simulink model "flightSimulation"  (R2018a)
settings: Solver=FixedStepAuto  StartTime=0  StopTime=end_time  FixedStep=0.005  RelTol=1e-3  EnableMultiTasking=on
values from neighbouring files (symbols this model uses):
  initPosLLA = [37.6287386167 -122.393391133 100]    [cmdh.mat]    (also in cmdyaw.mat)
  mass = 1.53    [cmdh.mat]    (also in cmdyaw.mat)
  Ts = 0.01    [cmdh.mat]    (also in cmdyaw.mat)
undefined symbols (not defined in the file or in its folder): B, Earth, ft, m, p_limits, s, sigbuilder_block, sw_turb, umax, umin, Vehicle, WGS84
libraries: simulink x23, aerolibactuator x15, dspswit3 x12, dspsrcs4 x10, dsparch4 x7, aerolibconvert2 x4, aerolibanimutils x2, qcatlib x2, aerolibfltsims x2, aerolibutil x2, shared6dof x1, aerolibtransform2 x1
(part 1 of 4)
settings Model: Creator=The MathWorks, Inc.  LastModifiedBy=mengc
settings SolverCC: AlgebraicLoopSolver=LineSearch  AutoInsertRateTranBlk=on
settings DataIOCC: LimitDataPoints=on  SaveFormat=Array  SaveOutput=off  DSMLogging=off  SaveTime=off
settings OptimizationCC: BlockReduction=off  BufferReuse=off  LifeSpan=inf
settings DebuggingCC: AlgebraicLoopMsg=none  UnderspecifiedInitializationDetection=Classic  MergeDetectMultiDrivingBlocksExec=none  UnconnectedInputMsg=none  UnconnectedOutputMsg=none  UnconnectedLineMsg=none  AllowSymbolicDim=off  SFUnexpectedBacktrackingDiag=warning  SFNoUnconditionalDefaultTransitionDiag=warning  SFExecutionAtInitializationDiag=none
settings HardwareCC: ProdBitPerPointer=32  ProdBitPerSizeT=32  ProdBitPerPtrDiffT=32  ProdLargestAtomicFloat=None  ProdIntDivRoundTo=Undefined  ProdEndianess=Unspecified  ProdWordSize=32  ProdHWDeviceType=32-bit Generic
settings ModelReferenceCC: PropagateSignalLabelsOutOfModel=off
settings CodeAppCC: StateflowObjectComments=on
settings GRTTargetCC: TargetLangStandard=C89/C90 (ANSI)  GeneratePreprocessorConditionals=Disable all
settings ConfigComp: CovMetricSettings=dw  CovHtmlReporting=on  CovSaveCumulativeToWorkspaceVar=on  CovSaveSingleToWorkspaceVar=on  CovExternalEMLEnable=off  CovSFcnEnable=off

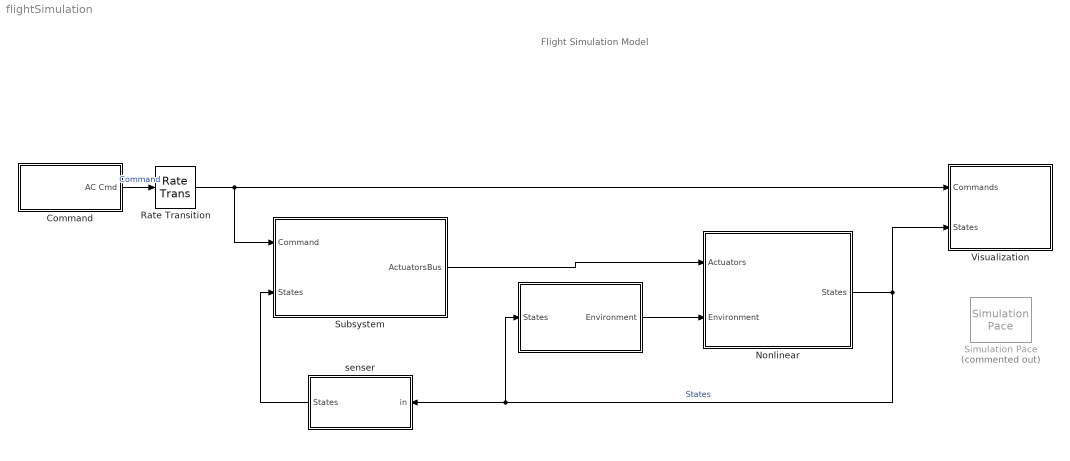
== system flightSimulation ==
  note: Flight Simulation Model
  " " : Subsystem
  Command : Subsystem  Variant=on
  Nonlinear : Subsystem  TreatAsAtomicUnit=on
      mask init:
      | vehicleNonlinearVars;
      settings: MinAlgLoopOccurrences=on
  Rate Transition : RateTransition  OutPortSampleTime=0.01
  Simulation Pace : aerolibanimutils/Simulation Pace  Commented=on  SimulationPace=1  SleepMode=MATLAB Thread  OutputPaceError=off  SampleTime=Ts
      settings: AttributesFormatString=%<SimulationPace> sec/sec
  Subsystem : Subsystem  Variant=on  VariantControl=Variant1
  Visualization : Subsystem
  senser : Subsystem
  wires:
  Nonlinear/1(States) -> senser/1(in), " "/1(States), Visualization/2(States)  "States"
  " "/1(Environment) -> Nonlinear/2(Environment)
  Command/1(AC Cmd) -> Rate Transition/1  "Command"
  Subsystem/1(ActuatorsBus) -> Nonlinear/1(Actuators)
  Rate Transition/1 -> Visualization/1(Commands), Subsystem/1("Command ")
  senser/1(States) -> Subsystem/2(States)

== system flightSimulation/  ==
  States : Inport  OutDataTypeStr=Bus: StatesBus
  Air Density : Constant  Value=1.225
  Air Temp : Constant  Value=273+15
  Bus Creator : BusCreator  Inputs=5  OutDataTypeStr=Bus: EnvironmentBus  NonVirtualBus=on
  Bus Creator1 : BusCreator  Inputs=4  OutDataTypeStr=Bus: AtmosphereBus  NonVirtualBus=on
  Gravity : Constant  Value=[0;0;9.788]
  Magnetic Field : Constant  Value=[0 0 0]
  Memory : Memory  InheritSampleTime=on
  Pressure : Constant  Value=101.3e3
  Speed of Sound : Constant  Value=340
  wind : Constant  Value=[0 0 0]
  Environment : Outport  OutDataTypeStr=Bus: EnvironmentBus
  wires:
  Pressure/1 -> Bus Creator1/3  "pressure"
  Magnetic Field/1 -> Bus Creator/3  "MagneticField_ned"
  Air Density/1 -> Bus Creator1/4  "air_density"
  Bus Creator1/1 -> Bus Creator/2  "AtmosphereBus"
  Gravity/1 -> Bus Creator/1  "Gravity_ned"
  Air Temp/1 -> Bus Creator1/1  "air_temp"
  Speed of Sound/1 -> Bus Creator1/2  "speed_sound"
  wind/1 -> Bus Creator/5  "Wind_ned"
  States/1 -> Memory/1  "StatesBus"
  Bus Creator/1 -> Environment/1  "EnvironmentBus"
  Memory/1 -> Bus Creator/4  "StatesBus"

== system flightSimulation/Command ==
  note: VSS_COMMAND = 0 will select Signal Builder
      | VSS_COMMAND =1 will select Joystick + Signal Builder
      | VSS_COMMAND = 2 will select pre-saved data from .mat file
      | VSS_COMMAND = 3 will select pre-saved data from a spreadsheet
  Data : Subsystem  VariantControl=VSS_COMMAND_PRESAVED
  Joystick : Subsystem  VariantControl=VSS_COMMAND_JOYSTICK
  Signal Builder : Subsystem  VariantControl=VSS_COMMAND_SIGBLDR
  Subsystem : Subsystem  VariantControl=VSS_COMMAND_user
  AC Cmd : Outport  OutDataTypeStr=Bus: CommandBus

== system flightSimulation/Nonlinear ==
  Actuators : Inport  OutDataTypeStr=Bus: ActuatorsBus
  Environment : Inport  Port=2  OutDataTypeStr=Bus: EnvironmentBus
  Plant : Subsystem
  States : Outport
  wires:
  Actuators/1 -> Plant/1(Actuators)  "ActuatorsBus"
  Environment/1 -> Plant/2(Environment)  "Environment"
  Plant/1(States) -> States/1

== system flightSimulation/Subsystem ==
  "Command " : Inport  OutDataTypeStr=Bus: CommandBus
  States : Inport  Port=2  OutDataTypeStr=Bus: StatesBus
  ADRC_allocator : Subsystem  VariantControl=controller==0
  ADRC_allocator1 : Subsystem  VariantControl=controller==1
  PID : Subsystem  VariantControl=controller==2
  PID_allocator : Subsystem  VariantControl=controller==3
  PID_allocator1 : Subsystem  VariantControl=controller==4
  ActuatorsBus : Outport  OutDataTypeStr=Bus: ActuatorsBus

== system flightSimulation/Visualization ==
  Commands : Inport
  States : Inport  Port=2
  Airspeed Indicator : Subsystem  DialogController=aeroblksHMICreateDDGDialog  IsWebBlock=on  mask(MWDashboardBlock){webBlockId=8420f0a9-3312-4f04-a723-760894642590, webBlockType=airspeedindicator, ShowInLibBrowser=on, ShowInitialText=on, HMISrcModelName=flightSimulation}
      mask prompts: webBlockId "WebBlock Id"; webBlockType "WebBlock Type"; HMISrcModelName "Source Model"
      mask help: Display aircraft airspeed in knots.
      mask Help: asbhmihelp('airspeedindicator')
      mask Display:
      | if strcmp(get_param(bdroot(gcb),'BlockDiagramType'), 'library')
      |  image([(matlabroot) '/toolbox/aeroblks/aeroblks/hmi/icons/AirspeedIndicatorIcon.svg'])
      | end
  Altimeter : Subsystem  DialogController=aeroblksHMICreateDDGDialog  IsWebBlock=on  mask(MWDashboardBlock){webBlockId=acc0ee33-6e2a-46f3-b359-bda7f19c378b, webBlockType=altimeter, ShowInLibBrowser=on, ShowInitialText=on, HMISrcModelName=flightSimulation}
      mask prompts: webBlockId "WebBlock Id"; webBlockType "WebBlock Type"; HMISrcModelName "Source Model"
      mask help: Display aircraft altitude in feet.
      mask Help: asbhmihelp('altimeter')
      mask Display:
      | if strcmp(get_param(bdroot(gcb),'BlockDiagramType'), 'library')
      |  image([(matlabroot) '/toolbox/aeroblks/aeroblks/hmi/icons/AltimeterIcon.svg'])
      | end
  Artificial Horizon : Subsystem  DialogController=aeroblksHMICreateDDGDialog  IsWebBlock=on  mask(MWDashboardBlock){webBlockId=e5cf728d-e454-405c-bb84-955fe1273f2a, webBlockType=artificialhorizon, ShowInLibBrowser=on, ShowInitialText=on, HMISrcModelName=flightSimulation}
      mask prompts: webBlockId "WebBlock Id"; webBlockType "WebBlock Type"; HMISrcModelName "Source Model"
      mask help: Display aircraft attitude relative to horizon. The two signal input vector contains roll and pitch.
      mask Help: asbhmihelp('artificialhorizon')
      mask Display:
      | if strcmp(get_param(bdroot(gcb),'BlockDiagramType'), 'library')
      |  image([(matlabroot) '/toolbox/aeroblks/aeroblks/hmi/icons/ArtificialHorizonIcon.svg'])
      | end
  Climb Rate Indicator : Subsystem  DialogController=aeroblksHMICreateDDGDialog  IsWebBlock=on  mask(MWDashboardBlock){webBlockId=da4b646e-398f-4414-b979-eb288c63e8d1, webBlockType=climbindicator, ShowInLibBrowser=on, ShowInitialText=on, HMISrcModelName=flightSimulation}
      mask prompts: webBlockId "WebBlock Id"; webBlockType "WebBlock Type"; HMISrcModelName "Source Model"
      mask help: Display aircraft climb rate in ft/min.
      mask Help: asbhmihelp('climbindicator')
      mask Display:
      | if strcmp(get_param(bdroot(gcb),'BlockDiagramType'), 'library')
      |  image([(matlabroot) '/toolbox/aeroblks/aeroblks/hmi/icons/ClimbIndicatorIcon.svg'])
      | end
  Extract Flight Instruments : Subsystem
  Heading Indicator : Subsystem  DialogController=aeroblksHMICreateDDGDialog  IsWebBlock=on  mask(MWDashboardBlock){webBlockId=33c4a518-f501-4d9d-9c87-ec3702c656b3, webBlockType=headingindicator, ShowInLibBrowser=on, ShowInitialText=on, HMISrcModelName=flightSimulation}
      mask prompts: webBlockId "WebBlock Id"; webBlockType "WebBlock Type"; HMISrcModelName "Source Model"
      mask help: Display aircraft heading with respect to North in degrees.
      mask Help: asbhmihelp('headingindicator')
      mask Display:
      | if strcmp(get_param(bdroot(gcb),'BlockDiagramType'), 'library')
      |  image([(matlabroot) '/toolbox/aeroblks/aeroblks/hmi/icons/HeadingIndicatorIcon.svg'])
      | end
  Visualization : Subsystem  Variant=on
  wires:
  Commands/1 -> Visualization/2(Commands)
  States/1 -> Visualization/1(States), Extract Flight Instruments/1(States)

== system flightSimulation/senser ==
  in : Inport  OutDataTypeStr=Bus: StatesBus
  Bus Creator5 : BusCreator  Inputs=9  OutDataTypeStr=Bus: StatesBus  NonVirtualBus=on
  Bus Selector1 : BusSelector  OutputSignals=V_body,Omega_body,Euler,Accel_body,dOmega_body,V_ned,X_ned,LLA,DCM_be
  Rate Transition2 : RateTransition  OutPortSampleTime=0.01
  noise : Subsystem
  States : Outport  OutDataTypeStr=Bus: StatesBus
  wires:
  Bus Selector1/1 -> Bus Creator5/1  "<V_body>"
  in/1 -> Bus Selector1/1
  Bus Selector1/7 -> Bus Creator5/7  "<X_ned>"
  Bus Selector1/8 -> Bus Creator5/8  "<LLA>"
  Bus Selector1/2 -> Bus Creator5/2  "<Omega_body>"
  Bus Selector1/9 -> Bus Creator5/9  "<DCM_be>"
  Bus Selector1/4 -> Bus Creator5/4  "<Accel_body>"
  Bus Selector1/5 -> Bus Creator5/5  "<dOmega_body>"
  Bus Selector1/6 -> Bus Creator5/6  "<V_ned>"
  Bus Selector1/3 -> noise/1(In1)  "<Euler>"
  Bus Creator5/1 -> Rate Transition2/1
  noise/1(Out1) -> Bus Creator5/3  "Euler"
  Rate Transition2/1 -> States/1

== system flightSimulation/Command/Data ==
  Bus Creator : BusCreator  Inputs=4  OutDataTypeStr=Bus: CommandBus  NonVirtualBus=on
  From Workspace : FromWorkspace  VariableName=cmdroll  SampleTime=0
  From Workspace1 : FromWorkspace  VariableName=cmdpitch  SampleTime=0
  From Workspace2 : FromWorkspace  VariableName=cmdyaw  SampleTime=0
  From Workspace3 : FromWorkspace  VariableName=cmdh  SampleTime=0
  Step : Step  Time=10  After=0.1  SampleTime=0
  Step1 : Step  Time=10  After=0  SampleTime=0
  Terminator : Terminator
  AC Cmd : Outport  OutDataTypeStr=Bus: CommandBus
  wires:
  Bus Creator/1 -> AC Cmd/1
  From Workspace1/1 -> Bus Creator/2  "pitch_cmd"
  From Workspace2/1 -> Bus Creator/3  "yaw_cmd"
  From Workspace3/1 -> Bus Creator/4  "throttle_cmd"
  From Workspace/1 -> Bus Creator/1  "roll_cmd"
  Step/1 -> Terminator/1

== system flightSimulation/Command/Joystick ==
  Bus Creator : BusCreator  Inputs=4  OutDataTypeStr=Bus: CommandBus  NonVirtualBus=on
  Pilot Joystick : aerolibanimutils/Pilot Joystick  JoystickID=Joystick1  OutputConfiguration=FourAxis  SampleTime=Ts
  AC Cmd : Outport  OutDataTypeStr=Bus: CommandBus
  wires:
  Pilot Joystick/4 -> Bus Creator/4  "throttle_cmd"
  Pilot Joystick/3 -> Bus Creator/3  "yaw_cmd"
  Pilot Joystick/2 -> Bus Creator/2  "pitch_cmd"
  Pilot Joystick/1 -> Bus Creator/1  "roll_cmd"
  Bus Creator/1 -> AC Cmd/1

== system flightSimulation/Command/Signal Builder ==
  Bus Creator : BusCreator  Inputs=4  OutDataTypeStr=Bus: CommandBus  NonVirtualBus=on
  N-Sample Switch : dspswit3/N-Sample Switch  N=200  reset=off  TriggerType=Rising edge  Ts=0.01
      settings: SourceProductName=DSP System Toolbox  SourceProductBaseCode=DS
  Pulse Generator : DiscretePulseGenerator  Amplitude=0.2  Period=300  PulseWidth=150  SampleTime=0.01
  Signal Builder : Subsystem  Tag=STV Subsys  LoadFcn=sigbuilder_block('load',[3 6 804 505.5 ]);  StartFcn=sigbuilder_block('start');  StopFcn=sigbuilder_block('stop');  ClipboardFcn=sigbuilder_block('clipboard');  mask(Sigbuilder block){tuvar=[0:10]}
      mask help: Simulink:masks:SigbuilderBlock_MD
      mask init:
      | if ~strcmp(get_param(bdroot(gcbh),'SimulationStatus'),'stopped') tuvar = sigbuilder_block('maskInit'); end
      settings: CopyFcn=sigbuilder_block('copy');  DeleteFcn=sigbuilder_block('delete');  ModelCloseFcn=sigbuilder_block('modelClose');  PreSaveFcn=sigbuilder_block('preSave');  PauseFcn=sigbuilder_block('pause');  ContinueFcn=sigbuilder_block('continue');  NameChangeFcn=sigbuilder_block('namechange');  OpenFcn=sigbuilder_block('open',[3 6 804 505.5 ]);  CloseFcn=sigbuilder_block('close');
      mask Display: plot(0, 0, 100, 100,[2, 2, 32, 32, 2], [68, 8, 8, 68, 68],[32, 2], [38, 38], [32, 19, 2],[53, 60, 44], [32, 17, 17, 2],[16, 16, 31, 31]);txt = getActiveGroup(gcbh);text(2, 100, txt,'verticalAlignment', 'top');
  Sine Wave : Sin  Amplitude=0.2  Frequency=2*pi/3  Samples=2000  SampleTime=0.01
  To Workspace : ToWorkspace  VariableName=simout  SaveFormat=Timeseries  SampleTime=-1
  roll_cmd : Step  Time=0  After=0  SampleTime=0
  throttle_cmd : Step  Time=0  After=0.5  SampleTime=0
  yaw_cmd : Step  Time=0  After=0  SampleTime=0
  AC Cmd : Outport  OutDataTypeStr=Bus: CommandBus
  wires:
  Bus Creator/1 -> AC Cmd/1
  Signal Builder/4(throttle_cmd) -> Bus Creator/4  "throttle_cmd"
  Signal Builder/2(picth_cmd) -> Bus Creator/2  "pitch_cmd"
  Signal Builder/3(yaw_cmd) -> Bus Creator/3  "yaw_cmd"
  Signal Builder/1(roll_cmd) -> Bus Creator/1  "roll_cmd"
  Pulse Generator/1 -> N-Sample Switch/2

== system flightSimulation/Command/Subsystem ==
  Bus Creator : BusCreator  Inputs=4  OutDataTypeStr=Bus: CommandBus  NonVirtualBus=on
  Signal Builder : Subsystem  Tag=STV Subsys  LoadFcn=sigbuilder_block('load',[0 30 1024.5 487.5 ]);  StartFcn=sigbuilder_block('start');  StopFcn=sigbuilder_block('stop');  ClipboardFcn=sigbuilder_block('clipboard');  mask(Sigbuilder block){tuvar=[0:10]}
      mask help: Simulink:masks:SigbuilderBlock_MD
      mask init:
      | if ~strcmp(get_param(bdroot(gcbh),'SimulationStatus'),'stopped') tuvar = sigbuilder_block('maskInit'); end
      settings: CopyFcn=sigbuilder_block('copy');  DeleteFcn=sigbuilder_block('delete');  ModelCloseFcn=sigbuilder_block('modelClose');  PreSaveFcn=sigbuilder_block('preSave');  PauseFcn=sigbuilder_block('pause');  ContinueFcn=sigbuilder_block('continue');  NameChangeFcn=sigbuilder_block('namechange');  OpenFcn=sigbuilder_block('open',[3 6 804 505.5 ]);  CloseFcn=sigbuilder_block('close');
      mask Display: plot(0, 0, 100, 100,[2, 2, 32, 32, 2], [68, 8, 8, 68, 68],[32, 2], [38, 38], [32, 19, 2],[53, 60, 44], [32, 17, 17, 2],[16, 16, 31, 31]);txt = getActiveGroup(gcbh);text(2, 100, txt,'verticalAlignment', 'top');
  Signal Builder1 : Subsystem  Tag=STV Subsys  LoadFcn=sigbuilder_block('load');  StartFcn=sigbuilder_block('start');  StopFcn=sigbuilder_block('stop');  ClipboardFcn=sigbuilder_block('clipboard');  mask(Sigbuilder block){tuvar=[0:10]}
      mask help: Simulink:masks:SigbuilderBlock_MD
      mask init:
      | if ~strcmp(get_param(bdroot(gcbh),'SimulationStatus'),'stopped') tuvar = sigbuilder_block('maskInit'); end
      settings: CopyFcn=sigbuilder_block('copy');  DeleteFcn=sigbuilder_block('delete');  ModelCloseFcn=sigbuilder_block('modelClose');  PreSaveFcn=sigbuilder_block('preSave');  PauseFcn=sigbuilder_block('pause');  ContinueFcn=sigbuilder_block('continue');  NameChangeFcn=sigbuilder_block('namechange');  OpenFcn=sigbuilder_block('open',[0 30 1024.5 487.5 ]);  CloseFcn=sigbuilder_block('close');
      mask Display: plot(0, 0, 100, 100,[2, 2, 32, 32, 2], [68, 8, 8, 68, 68],[32, 2], [38, 38], [32, 19, 2],[53, 60, 44], [32, 17, 17, 2],[16, 16, 31, 31]);txt = getActiveGroup(gcbh);text(2, 100, txt,'verticalAlignment', 'top');
  AC Cmd : Outport  OutDataTypeStr=Bus: CommandBus
  wires:
  Bus Creator/1 -> AC Cmd/1
  Signal Builder/1(roll_cmd) -> Bus Creator/1  "roll_cmd"
  Signal Builder/2(picth_cmd) -> Bus Creator/2  "pitch_cmd"
  Signal Builder/3(yaw_cmd) -> Bus Creator/3  "yaw_cmd"
  Signal Builder/4(throttle_cmd) -> Bus Creator/4  "throttle_cmd"

== system flightSimulation/Nonlinear/Plant ==
  Actuators : Inport  OutDataTypeStr=Bus: ActuatorsBus
  Environment : Inport  Port=2  OutDataTypeStr=Bus: EnvironmentBus
  6DOF (Quaternion) : shared6dof/6DOF (Euler Angles)  units=Metric (MKS)  mtype=Fixed  rep=Euler Angles  xme_0=initPosNED  Vm_0=initVb  eul_0=initEuler  pm_0=initAngRates  mass_0=mass  mass_e=0.5  mass_f=2.0  inertia=inertia  inertia_e=eye(3)  inertia_f=2*eye(3)  k_quat=Vehicle.Nonlinear.Nonlinear.SixDOF.quatGain  vre_flag=on  abi_flag=on  aMode=aMode
      settings: SourceProductBaseCode=AE
  Bus setup : Subsystem
  Position on Earth : Subsystem  Priority=1  TreatAsAtomicUnit=on
  Subsystem : Subsystem
  Subsystem1 : Subsystem
  Sum : Sum  Inputs=|++
  Terminator : Terminator
  States : Outport  OutDataTypeStr=Bus: StatesBus
  wires:
  Position on Earth/1(LLA) -> Bus setup/1(LLA)
  6DOF (Quaternion)/8 -> Terminator/1
  6DOF (Quaternion)/1 -> Bus setup/2(V_ned)
  6DOF (Quaternion)/2 -> Position on Earth/1(Xe), Bus setup/3(X_ned)
  6DOF (Quaternion)/9 -> Bus setup/9(Accel_b)
  6DOF (Quaternion)/5 -> Bus setup/6(V_b)
  6DOF (Quaternion)/7 -> Bus setup/8(dOmega_b)
  6DOF (Quaternion)/4 -> Bus setup/5(DCM_be)  "Rn2b"
  Bus setup/1(States) -> States/1  "StatesBus"
  Environment/1 -> Subsystem/2(EnvironmentBus), Subsystem1/2(In2)  "EnvironmentBus"
  Subsystem/1(Out1) -> 6DOF (Quaternion)/1
  Actuators/1 -> Subsystem1/1(In1), Subsystem/1(ActuatorsBus)  "ActuatorsBus"
  Subsystem1/1(Out1) -> Sum/1
  Sum/1 -> 6DOF (Quaternion)/2
  6DOF (Quaternion)/6 -> Bus setup/7(Omega_b)
  6DOF (Quaternion)/3 -> Bus setup/4(Euler)

== system flightSimulation/Subsystem/ADRC_allocator ==
  Command : Inport
  States : Inport  Port=2  OutDataTypeStr=Bus: StatesBus
  Add : Sum
  Bus Creator : BusCreator  Inputs=5  OutDataTypeStr=Bus: ActuatorsBus
  Bus Selector : BusSelector  OutputSignals=roll_cmd,pitch_cmd,yaw_cmd,throttle_cmd
  Bus Selector1 : BusSelector  OutputSignals=<Euler>,Omega_body,X_ned,V_ned
  Constant : Constant  Value=-9.788
  Constant1 : Constant  Value=1225
  Demux : Demux  Outputs=3
  Demux2 : Demux  Outputs=3
  Demux3 : Demux  Outputs=3
  Demux4 : Demux  Outputs=2
  Demux5 : Demux  Outputs=2
  MATLAB Function : MATLAB Function  TreatAsAtomicUnit=on
  MATLAB Function2 : MATLAB Function  TreatAsAtomicUnit=on
  MATLAB Function3 : MATLAB Function  TreatAsAtomicUnit=on
  N-Sample Switch : dspswit3/N-Sample Switch  N=3  reset=off  TriggerType=Rising edge  Ts=0.01
      settings: SourceProductName=DSP System Toolbox  SourceProductBaseCode=DS
  PID Controller (2DOF)7 : simulink/Continuous/PID Controller (2DOF)  Controller=PID  TimeDomain=Discrete-time  SampleTime=-1  IntegratorMethod=Forward Euler  FilterMethod=Forward Euler  Form=Parallel  UseFilter=on  ControllerParametersSource=internal  P=2.1  I=0.2  D=2.1  N=100  b=1  c=1  InitialConditionSource=internal  InitialConditionForIntegrator=0  InitialConditionForFilter=0  ExternalReset=none  LimitOutput=off  UpperSaturationLimit=inf  LowerSaturationLimit=-inf  LinearizeAsGain=on  AntiWindupMode=none  Kb=1  TrackingMode=off  Kt=1  PParamMin=[]  PParamMax=[]  IParamMin=[]  IParamMax=[]  DParamMin=[]  DParamMax=[]  NParamMin=[]  NParamMax=[]  bParamMin=[]  bParamMax=[]  cParamMin=[]  cParamMax=[]  KbParamMin=[]  KbParamMax=[]  KtParamMin=[]  KtParamMax=[]  POutMin=[]  POutMax=[]  IOutMin=[]  IOutMax=[]  DOutMin=[]  DOutMax=[]  NOutMin=[]  NOutMax=[]  bOutMin=[]  bOutMax=[]  cOutMin=[]  cOutMax=[]  KbOutMin=[]  KbOutMax=[]  KtOutMin=[]  KtOutMax=[]  IntegratorOutMin=[]  IntegratorOutMax=[]  FilterOutMin=[]  FilterOutMax=[]  SumOutMin=[]  SumOutMax=[]  Sum1OutMin=[]  Sum1OutMax=[]  Sum2OutMin=[]  Sum2OutMax=[]  Sum3OutMin=[]  Sum3OutMax=[]  SumI1OutMin=[]  SumI1OutMax=[]  SumI2OutMin=[]  SumI2OutMax=[]  SumI3OutMin=[]  SumI3OutMax=[]  SumDOutMin=[]  SumDOutMax=[]  SaturationOutMin=[]  SaturationOutMax=[]  IntegratorContinuousStateAttributes=''  IntegratorStateMustResolveToSignalObject=off  IntegratorRTWStateStorageClass=Auto  FilterContinuousStateAttributes=''  FilterStateMustResolveToSignalObject=off  FilterRTWStateStorageClass=Auto  DifferentiatorICPrevScaledInput=0  DifferentiatorOutMin=[]  DifferentiatorOutMax=[]  FilterDiffOutCoefMin=[]  FilterDiffOutCoefMax=[]  SumDenOutMin=[]  SumDenOutMax=[]  SumNumOutMin=[]  SumNumOutMax=[]  ReciprocalOutMin=[]  ReciprocalOutMax=[]  DivideOutMin=[]  DivideOutMax=[]  TunerSelectOption=Transfer Function Based (PID Tuner App)
  S-Function : S-Function  FunctionName=s_yawTD  SFunctionDeploymentMode=off  EnableBusSupport=off
  S-Function1 : S-Function  FunctionName=s_TD  SFunctionDeploymentMode=off  EnableBusSupport=off
  S-Function2 : S-Function  FunctionName=s_TD  SFunctionDeploymentMode=off  EnableBusSupport=off
  Saturation : Saturate  UpperLimit=9.788  LowerLimit=-9.788
  Subsystem : Subsystem
  Subsystem2 : Subsystem
  TD : Demux  Outputs=2
  Terminator2 : Terminator
  Terminator3 : Terminator
  Unit Delay1 : UnitDelay  SampleTime=-1
  舵机偏角输入eso : Subsystem
  ActuatorsBus : Outport  OutDataTypeStr=Bus: ActuatorsBus
  wires:
  PID Controller (2DOF)7/1 -> Saturation/1
  Bus Selector1/2 -> 舵机偏角输入eso/6(<pqr>)  "<Omega_body>"
  Demux3/2 -> Terminator2/1
  Demux/2 -> Subsystem/1(q)
  Demux3/1 -> Terminator3/1
  Bus Selector/4 -> PID Controller (2DOF)7/1  "<throttle_cmd>"
  Command/1 -> Bus Selector/1
  Bus Creator/1 -> ActuatorsBus/1  "ActuatorsBus"
  Constant1/1 -> N-Sample Switch/1
  Subsystem/1(speed) -> N-Sample Switch/2  "speed"
  N-Sample Switch/1 -> Bus Creator/5  "speed"
  Demux3/3 -> PID Controller (2DOF)7/2  "h"
  States/1 -> Unit Delay1/1
  Unit Delay1/1 -> Bus Selector1/1
  Add/1 -> Subsystem/3(In3)  "a_t"
  Constant/1 -> Add/1
  Saturation/1 -> Add/2
  Demux/1 -> Subsystem/2(p)
  Subsystem2/1(c1) -> Bus Creator/1
  Subsystem2/3(c3) -> Bus Creator/3
  Subsystem2/2(c2) -> Bus Creator/2
  Bus Selector1/3 -> Demux3/1  "<X_ned>"
  Subsystem2/4(c4) -> Bus Creator/4
  Bus Selector1/1 -> 舵机偏角输入eso/5(<Euler>), Demux/1  "<<Euler>>"
  舵机偏角输入eso/7(反馈) -> Demux2/1
  S-Function/1 -> Demux4/1
  Demux4/1 -> MATLAB Function/1(x1_d)  "偏航_跟踪"
  Demux4/2 -> MATLAB Function/2(x2_d)
  Bus Selector/3 -> S-Function/1  "<yaw_cmd>"
  S-Function1/1 -> Demux5/1
  Demux5/2 -> MATLAB Function2/2(x2_d)
  Demux5/1 -> MATLAB Function2/1(x1_d)  "俯仰_跟踪"
  TD/1 -> MATLAB Function3/1(x1_d)  "滚转_跟踪"
  TD/2 -> MATLAB Function3/2(x2_d)
  S-Function2/1 -> TD/1
  Bus Selector/1 -> S-Function2/1  "<roll_cmd>"
  Bus Selector/2 -> S-Function1/1  "<pitch_cmd>"
  MATLAB Function/1(u_r) -> Subsystem2/3(u_3)  "ur"
  MATLAB Function3/1(u_p) -> Subsystem2/1(u_1)  "up"
  MATLAB Function2/1(u_q) -> Subsystem2/2(u_2)  "uq"
  舵机偏角输入eso/1(滚转估计) -> MATLAB Function3/3(x1)
  舵机偏角输入eso/2(俯仰估计) -> MATLAB Function2/3(x1)
  舵机偏角输入eso/3(偏航估计) -> MATLAB Function/3(x1)
  舵机偏角输入eso/4(P估计) -> MATLAB Function3/4(x2)
  舵机偏角输入eso/5(q估计) -> MATLAB Function2/4(x2)
  舵机偏角输入eso/6(r估计) -> MATLAB Function/4(x2)
  Demux2/1 -> Subsystem2/4(u_4)  "dp"
  Demux2/2 -> Subsystem2/5(u_5)  "dq"
  Demux2/3 -> Subsystem2/6(u_6)  "dr"
  Subsystem2/5(c5) -> 舵机偏角输入eso/1(c1)
  Subsystem2/6(c6) -> 舵机偏角输入eso/2(c2)
  Subsystem2/7(c7) -> 舵机偏角输入eso/3(c3)
  Subsystem2/8(c8) -> 舵机偏角输入eso/4(c4)

== system flightSimulation/Subsystem/ADRC_allocator1 ==
  Command : Inport
  States : Inport  Port=2  OutDataTypeStr=Bus: StatesBus
  Add : Sum
  Bus Creator : BusCreator  Inputs=5  OutDataTypeStr=Bus: ActuatorsBus
  Bus Selector : BusSelector  OutputSignals=roll_cmd,pitch_cmd,yaw_cmd,throttle_cmd
  Bus Selector1 : BusSelector  OutputSignals=Euler,Omega_body,X_ned
  Constant : Constant  Value=-9.788
  Constant1 : Constant  Value=1225  SampleTime=0.005
  Demux : Demux  Outputs=3
  Demux2 : Demux  Outputs=3
  Demux3 : Demux  Outputs=3
  Demux4 : Demux  Outputs=2
  Demux5 : Demux  Outputs=2
  MATLAB Function : MATLAB Function  TreatAsAtomicUnit=on
  MATLAB Function2 : MATLAB Function  TreatAsAtomicUnit=on
  MATLAB Function3 : MATLAB Function  TreatAsAtomicUnit=on
  N-Sample Switch : dspswit3/N-Sample Switch  N=10  reset=off  TriggerType=Rising edge  Ts=0.005
      settings: SourceProductName=DSP System Toolbox  SourceProductBaseCode=DS
  PID Controller (2DOF)7 : simulink/Continuous/PID Controller (2DOF)  Controller=PID  TimeDomain=Discrete-time  SampleTime=0.01  IntegratorMethod=Forward Euler  FilterMethod=Forward Euler  Form=Parallel  UseFilter=on  ControllerParametersSource=internal  P=2.1  I=0.2  D=2.1  N=100  b=1  c=1  InitialConditionSource=internal  InitialConditionForIntegrator=0  InitialConditionForFilter=0  ExternalReset=none  LimitOutput=off  UpperSaturationLimit=inf  LowerSaturationLimit=-inf  LinearizeAsGain=on  AntiWindupMode=none  Kb=1  TrackingMode=off  Kt=1  PParamMin=[]  PParamMax=[]  IParamMin=[]  IParamMax=[]  DParamMin=[]  DParamMax=[]  NParamMin=[]  NParamMax=[]  bParamMin=[]  bParamMax=[]  cParamMin=[]  cParamMax=[]  KbParamMin=[]  KbParamMax=[]  KtParamMin=[]  KtParamMax=[]  POutMin=[]  POutMax=[]  IOutMin=[]  IOutMax=[]  DOutMin=[]  DOutMax=[]  NOutMin=[]  NOutMax=[]  bOutMin=[]  bOutMax=[]  cOutMin=[]  cOutMax=[]  KbOutMin=[]  KbOutMax=[]  KtOutMin=[]  KtOutMax=[]  IntegratorOutMin=[]  IntegratorOutMax=[]  FilterOutMin=[]  FilterOutMax=[]  SumOutMin=[]  SumOutMax=[]  Sum1OutMin=[]  Sum1OutMax=[]  Sum2OutMin=[]  Sum2OutMax=[]  Sum3OutMin=[]  Sum3OutMax=[]  SumI1OutMin=[]  SumI1OutMax=[]  SumI2OutMin=[]  SumI2OutMax=[]  SumI3OutMin=[]  SumI3OutMax=[]  SumDOutMin=[]  SumDOutMax=[]  SaturationOutMin=[]  SaturationOutMax=[]  IntegratorContinuousStateAttributes=''  IntegratorStateMustResolveToSignalObject=off  IntegratorRTWStateStorageClass=Auto  FilterContinuousStateAttributes=''  FilterStateMustResolveToSignalObject=off  FilterRTWStateStorageClass=Auto  DifferentiatorICPrevScaledInput=0  DifferentiatorOutMin=[]  DifferentiatorOutMax=[]  FilterDiffOutCoefMin=[]  FilterDiffOutCoefMax=[]  SumDenOutMin=[]  SumDenOutMax=[]  SumNumOutMin=[]  SumNumOutMax=[]  ReciprocalOutMin=[]  ReciprocalOutMax=[]  DivideOutMin=[]  DivideOutMax=[]  TunerSelectOption=Transfer Function Based (PID Tuner App)
  S-Function : S-Function  FunctionName=s_yawTD  SFunctionDeploymentMode=off  EnableBusSupport=off
  S-Function1 : S-Function  FunctionName=s_TD  SFunctionDeploymentMode=off  EnableBusSupport=off
  S-Function2 : S-Function  FunctionName=s_TD  SFunctionDeploymentMode=off  EnableBusSupport=off
  Saturation : Saturate  UpperLimit=9.788  LowerLimit=-9.788
  Subsystem : Subsystem
  Subsystem2 : Subsystem
  TD : Demux  Outputs=2
  Terminator2 : Terminator
  Terminator3 : Terminator
  input noise : Subsystem
  舵机偏角输入eso : Subsystem
  ActuatorsBus : Outport  OutDataTypeStr=Bus: ActuatorsBus
  wires:
  PID Controller (2DOF)7/1 -> Saturation/1
  Bus Selector1/2 -> 舵机偏角输入eso/3(<pqr>)  "<Omega_body>"
  Demux3/2 -> Terminator2/1
  Demux/2 -> Subsystem/1(q)
  Demux3/1 -> Terminator3/1
  Bus Selector/4 -> PID Controller (2DOF)7/1  "<throttle_cmd>"
  Command/1 -> Bus Selector/1
  Bus Creator/1 -> ActuatorsBus/1  "ActuatorsBus"
  Constant1/1 -> N-Sample Switch/1
  Subsystem/1(speed) -> N-Sample Switch/2  "speed"
  N-Sample Switch/1 -> Bus Creator/5  "speed"
  Demux3/3 -> PID Controller (2DOF)7/2  "h"
  Add/1 -> Subsystem/3(In3)  "a_t"
  Constant/1 -> Add/1
  Saturation/1 -> Add/2
  Demux/1 -> Subsystem/2(p)
  Subsystem2/1(c1) -> Bus Creator/1
  Subsystem2/3(c3) -> Bus Creator/3
  Subsystem2/2(c2) -> Bus Creator/2
  Bus Selector1/3 -> Demux3/1  "<X_ned>"
  Subsystem2/4(c4) -> Bus Creator/4
  S-Function/1 -> Demux4/1
  Demux4/1 -> MATLAB Function/1(x1_d)  "偏航_跟踪"
  Demux4/2 -> MATLAB Function/2(x2_d)
  Bus Selector/3 -> input noise/3(In3)  "<yaw_cmd>"
  S-Function1/1 -> Demux5/1
  Demux5/2 -> MATLAB Function2/2(x2_d)
  Demux5/1 -> MATLAB Function2/1(x1_d)  "俯仰_跟踪"
  TD/1 -> MATLAB Function3/1(x1_d)  "滚转_跟踪"
  TD/2 -> MATLAB Function3/2(x2_d)
  S-Function2/1 -> TD/1
  Bus Selector/1 -> input noise/1(In1)  "<roll_cmd>"
  Bus Selector/2 -> input noise/2(In2)  "<pitch_cmd>"
  MATLAB Function/1(u_r) -> Subsystem2/3(u_3)  "ur"
  MATLAB Function3/1(u_p) -> Subsystem2/1(u_1)  "up"
  MATLAB Function2/1(u_q) -> Subsystem2/2(u_2)  "uq"
  舵机偏角输入eso/1(滚转估计) -> MATLAB Function3/3(x1)
  舵机偏角输入eso/2(俯仰估计) -> MATLAB Function2/3(x1)
  舵机偏角输入eso/3(偏航估计) -> MATLAB Function/3(x1)
  舵机偏角输入eso/4(P估计) -> MATLAB Function3/4(x2)
  舵机偏角输入eso/5(q估计) -> MATLAB Function2/4(x2)
  舵机偏角输入eso/6(r估计) -> MATLAB Function/4(x2)
  Demux2/1 -> Subsystem2/4(u_4)  "dp"
  Demux2/2 -> Subsystem2/5(u_5)  "dq"
  Demux2/3 -> Subsystem2/6(u_6)  "dr"
  Subsystem2/5(c5) -> 舵机偏角输入eso/1(c1)
  舵机偏角输入eso/7(反馈) -> Demux2/1
  States/1 -> Bus Selector1/1
  Bus Selector1/1 -> Demux/1, 舵机偏角输入eso/2(<Euler>)  "<Euler>"
  input noise/1(Out1) -> S-Function2/1
  input noise/2(Out2) -> S-Function1/1
  input noise/3(Out3) -> S-Function/1

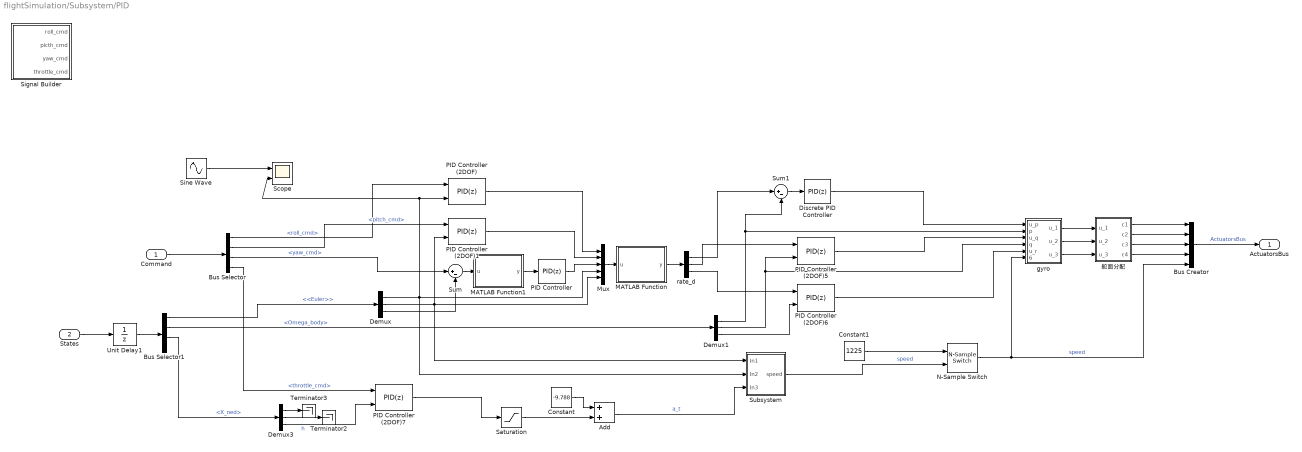
== system flightSimulation/Subsystem/PID ==
  Command : Inport
  States : Inport  Port=2  OutDataTypeStr=Bus: StatesBus
  Add : Sum
  Bus Creator : BusCreator  Inputs=5  OutDataTypeStr=Bus: ActuatorsBus
  Bus Selector : BusSelector  OutputSignals=roll_cmd,pitch_cmd,yaw_cmd,throttle_cmd
  Bus Selector1 : BusSelector  OutputSignals=<Euler>,Omega_body,X_ned,V_ned
  Constant : Constant  Value=-9.788
  Constant1 : Constant  Value=1225
  Demux : Demux  Outputs=3
  Demux1 : Demux  Outputs=3
  Demux3 : Demux  Outputs=3
  Discrete PID Controller : simulink/Continuous/PID Controller  Controller=PID  TimeDomain=Discrete-time  SampleTime=-1  IntegratorMethod=Forward Euler  FilterMethod=Forward Euler  Form=Parallel  UseFilter=on  ControllerParametersSource=internal  P=0.4  I=0.1  D=0  N=100  InitialConditionSource=internal  InitialConditionForIntegrator=0  InitialConditionForFilter=0  ExternalReset=none  LimitOutput=off  UpperSaturationLimit=inf  LowerSaturationLimit=-inf  LinearizeAsGain=off  AntiWindupMode=none  Kb=1  TrackingMode=off  Kt=1  PParamMin=[]  PParamMax=[]  IParamMin=[]  IParamMax=[]  DParamMin=[]  DParamMax=[]  NParamMin=[]  NParamMax=[]  KbParamMin=[]  KbParamMax=[]  KtParamMin=[]  KtParamMax=[]  POutMin=[]  POutMax=[]  IOutMin=[]  IOutMax=[]  DOutMin=[]  DOutMax=[]  NOutMin=[]  NOutMax=[]  KbOutMin=[]  KbOutMax=[]  KtOutMin=[]  KtOutMax=[]  IntegratorOutMin=[]  IntegratorOutMax=[]  FilterOutMin=[]  FilterOutMax=[]  SumOutMin=[]  SumOutMax=[]  SumI1OutMin=[]  SumI1OutMax=[]  SumI2OutMin=[]  SumI2OutMax=[]  SumI3OutMin=[]  SumI3OutMax=[]  SumDOutMin=[]  SumDOutMax=[]  SaturationOutMin=[]  SaturationOutMax=[]  IntegratorContinuousStateAttributes=''  IntegratorStateMustResolveToSignalObject=off  IntegratorRTWStateStorageClass=Auto  FilterContinuousStateAttributes=''  FilterStateMustResolveToSignalObject=off  FilterRTWStateStorageClass=Auto  DifferentiatorICPrevScaledInput=0  DifferentiatorOutMin=[]  DifferentiatorOutMax=[]  FilterDiffOutCoefMin=[]  FilterDiffOutCoefMax=[]  SumDenOutMin=[]  SumDenOutMax=[]  SumNumOutMin=[]  SumNumOutMax=[]  ReciprocalOutMin=[]  ReciprocalOutMax=[]  DivideOutMin=[]  DivideOutMax=[]  TunerSelectOption=Transfer Function Based (PID Tuner App)
  MATLAB Function : MATLAB Function  TreatAsAtomicUnit=on
  MATLAB Function1 : MATLAB Function  TreatAsAtomicUnit=on
  Mux : Mux  Inputs=5
  N-Sample Switch : dspswit3/N-Sample Switch  N=3  reset=off  TriggerType=Rising edge  Ts=0.01
      settings: SourceProductName=DSP System Toolbox  SourceProductBaseCode=DS
  PID Controller : simulink/Continuous/PID Controller  Controller=PID  TimeDomain=Discrete-time  SampleTime=-1  IntegratorMethod=Forward Euler  FilterMethod=Forward Euler  Form=Parallel  UseFilter=on  ControllerParametersSource=internal  P=5  I=0  D=0  N=100  InitialConditionSource=internal  InitialConditionForIntegrator=0  InitialConditionForFilter=0  ExternalReset=none  LimitOutput=off  UpperSaturationLimit=inf  LowerSaturationLimit=-inf  LinearizeAsGain=on  AntiWindupMode=none  Kb=1  TrackingMode=off  Kt=1  PParamMin=[]  PParamMax=[]  IParamMin=[]  IParamMax=[]  DParamMin=[]  DParamMax=[]  NParamMin=[]  NParamMax=[]  KbParamMin=[]  KbParamMax=[]  KtParamMin=[]  KtParamMax=[]  POutMin=[]  POutMax=[]  IOutMin=[]  IOutMax=[]  DOutMin=[]  DOutMax=[]  NOutMin=[]  NOutMax=[]  KbOutMin=[]  KbOutMax=[]  KtOutMin=[]  KtOutMax=[]  IntegratorOutMin=[]  IntegratorOutMax=[]  FilterOutMin=[]  FilterOutMax=[]  SumOutMin=[]  SumOutMax=[]  SumI1OutMin=[]  SumI1OutMax=[]  SumI2OutMin=[]  SumI2OutMax=[]  SumI3OutMin=[]  SumI3OutMax=[]  SumDOutMin=[]  SumDOutMax=[]  SaturationOutMin=[]  SaturationOutMax=[]  IntegratorContinuousStateAttributes=''  IntegratorStateMustResolveToSignalObject=off  IntegratorRTWStateStorageClass=Auto  FilterContinuousStateAttributes=''  FilterStateMustResolveToSignalObject=off  FilterRTWStateStorageClass=Auto  DifferentiatorICPrevScaledInput=0  DifferentiatorOutMin=[]  DifferentiatorOutMax=[]  FilterDiffOutCoefMin=[]  FilterDiffOutCoefMax=[]  SumDenOutMin=[]  SumDenOutMax=[]  SumNumOutMin=[]  SumNumOutMax=[]  ReciprocalOutMin=[]  ReciprocalOutMax=[]  DivideOutMin=[]  DivideOutMax=[]  TunerSelectOption=Transfer Function Based (PID Tuner App)
  PID Controller (2DOF) : simulink/Continuous/PID Controller (2DOF)  Controller=PID  TimeDomain=Discrete-time  SampleTime=-1  IntegratorMethod=Forward Euler  FilterMethod=Forward Euler  Form=Parallel  UseFilter=on  ControllerParametersSource=internal  P=7  I=0  D=0  N=100  b=1  c=1  InitialConditionSource=internal  InitialConditionForIntegrator=0  InitialConditionForFilter=0  ExternalReset=none  LimitOutput=off  UpperSaturationLimit=inf  LowerSaturationLimit=-inf  LinearizeAsGain=on  AntiWindupMode=none  Kb=1  TrackingMode=off  Kt=1  PParamMin=[]  PParamMax=[]  IParamMin=[]  IParamMax=[]  DParamMin=[]  DParamMax=[]  NParamMin=[]  NParamMax=[]  bParamMin=[]  bParamMax=[]  cParamMin=[]  cParamMax=[]  KbParamMin=[]  KbParamMax=[]  KtParamMin=[]  KtParamMax=[]  POutMin=[]  POutMax=[]  IOutMin=[]  IOutMax=[]  DOutMin=[]  DOutMax=[]  NOutMin=[]  NOutMax=[]  bOutMin=[]  bOutMax=[]  cOutMin=[]  cOutMax=[]  KbOutMin=[]  KbOutMax=[]  KtOutMin=[]  KtOutMax=[]  IntegratorOutMin=[]  IntegratorOutMax=[]  FilterOutMin=[]  FilterOutMax=[]  SumOutMin=[]  SumOutMax=[]  Sum1OutMin=[]  Sum1OutMax=[]  Sum2OutMin=[]  Sum2OutMax=[]  Sum3OutMin=[]  Sum3OutMax=[]  SumI1OutMin=[]  SumI1OutMax=[]  SumI2OutMin=[]  SumI2OutMax=[]  SumI3OutMin=[]  SumI3OutMax=[]  SumDOutMin=[]  SumDOutMax=[]  SaturationOutMin=[]  SaturationOutMax=[]  IntegratorContinuousStateAttributes=''  IntegratorStateMustResolveToSignalObject=off  IntegratorRTWStateStorageClass=Auto  FilterContinuousStateAttributes=''  FilterStateMustResolveToSignalObject=off  FilterRTWStateStorageClass=Auto  DifferentiatorICPrevScaledInput=0  DifferentiatorOutMin=[]  DifferentiatorOutMax=[]  FilterDiffOutCoefMin=[]  FilterDiffOutCoefMax=[]  SumDenOutMin=[]  SumDenOutMax=[]  SumNumOutMin=[]  SumNumOutMax=[]  ReciprocalOutMin=[]  ReciprocalOutMax=[]  DivideOutMin=[]  DivideOutMax=[]  TunerSelectOption=Transfer Function Based (PID Tuner App)
  PID Controller (2DOF)1 : simulink/Continuous/PID Controller (2DOF)  Controller=PID  TimeDomain=Discrete-time  SampleTime=-1  IntegratorMethod=Forward Euler  FilterMethod=Forward Euler  Form=Parallel  UseFilter=on  ControllerParametersSource=internal  P=7  I=0  D=0  N=100  b=1  c=1  InitialConditionSource=internal  InitialConditionForIntegrator=0  InitialConditionForFilter=0  ExternalReset=none  LimitOutput=off  UpperSaturationLimit=inf  LowerSaturationLimit=-inf  LinearizeAsGain=on  AntiWindupMode=none  Kb=1  TrackingMode=off  Kt=1  PParamMin=[]  PParamMax=[]  IParamMin=[]  IParamMax=[]  DParamMin=[]  DParamMax=[]  NParamMin=[]  NParamMax=[]  bParamMin=[]  bParamMax=[]  cParamMin=[]  cParamMax=[]  KbParamMin=[]  KbParamMax=[]  KtParamMin=[]  KtParamMax=[]  POutMin=[]  POutMax=[]  IOutMin=[]  IOutMax=[]  DOutMin=[]  DOutMax=[]  NOutMin=[]  NOutMax=[]  bOutMin=[]  bOutMax=[]  cOutMin=[]  cOutMax=[]  KbOutMin=[]  KbOutMax=[]  KtOutMin=[]  KtOutMax=[]  IntegratorOutMin=[]  IntegratorOutMax=[]  FilterOutMin=[]  FilterOutMax=[]  SumOutMin=[]  SumOutMax=[]  Sum1OutMin=[]  Sum1OutMax=[]  Sum2OutMin=[]  Sum2OutMax=[]  Sum3OutMin=[]  Sum3OutMax=[]  SumI1OutMin=[]  SumI1OutMax=[]  SumI2OutMin=[]  SumI2OutMax=[]  SumI3OutMin=[]  SumI3OutMax=[]  SumDOutMin=[]  SumDOutMax=[]  SaturationOutMin=[]  SaturationOutMax=[]  IntegratorContinuousStateAttributes=''  IntegratorStateMustResolveToSignalObject=off  IntegratorRTWStateStorageClass=Auto  FilterContinuousStateAttributes=''  FilterStateMustResolveToSignalObject=off  FilterRTWStateStorageClass=Auto  DifferentiatorICPrevScaledInput=0  DifferentiatorOutMin=[]  DifferentiatorOutMax=[]  FilterDiffOutCoefMin=[]  FilterDiffOutCoefMax=[]  SumDenOutMin=[]  SumDenOutMax=[]  SumNumOutMin=[]  SumNumOutMax=[]  ReciprocalOutMin=[]  ReciprocalOutMax=[]  DivideOutMin=[]  DivideOutMax=[]  TunerSelectOption=Transfer Function Based (PID Tuner App)
  PID Controller (2DOF)5 : simulink/Continuous/PID Controller (2DOF)  Controller=PID  TimeDomain=Discrete-time  SampleTime=-1  IntegratorMethod=Forward Euler  FilterMethod=Forward Euler  Form=Parallel  UseFilter=on  ControllerParametersSource=internal  P=0.4  I=0.1  D=0  N=100  b=1  c=1  InitialConditionSource=internal  InitialConditionForIntegrator=0  InitialConditionForFilter=0  ExternalReset=none  LimitOutput=off  UpperSaturationLimit=inf  LowerSaturationLimit=-inf  LinearizeAsGain=on  AntiWindupMode=none  Kb=1  TrackingMode=off  Kt=1  PParamMin=[]  PParamMax=[]  IParamMin=[]  IParamMax=[]  DParamMin=[]  DParamMax=[]  NParamMin=[]  NParamMax=[]  bParamMin=[]  bParamMax=[]  cParamMin=[]  cParamMax=[]  KbParamMin=[]  KbParamMax=[]  KtParamMin=[]  KtParamMax=[]  POutMin=[]  POutMax=[]  IOutMin=[]  IOutMax=[]  DOutMin=[]  DOutMax=[]  NOutMin=[]  NOutMax=[]  bOutMin=[]  bOutMax=[]  cOutMin=[]  cOutMax=[]  KbOutMin=[]  KbOutMax=[]  KtOutMin=[]  KtOutMax=[]  IntegratorOutMin=[]  IntegratorOutMax=[]  FilterOutMin=[]  FilterOutMax=[]  SumOutMin=[]  SumOutMax=[]  Sum1OutMin=[]  Sum1OutMax=[]  Sum2OutMin=[]  Sum2OutMax=[]  Sum3OutMin=[]  Sum3OutMax=[]  SumI1OutMin=[]  SumI1OutMax=[]  SumI2OutMin=[]  SumI2OutMax=[]  SumI3OutMin=[]  SumI3OutMax=[]  SumDOutMin=[]  SumDOutMax=[]  SaturationOutMin=[]  SaturationOutMax=[]  IntegratorContinuousStateAttributes=''  IntegratorStateMustResolveToSignalObject=off  IntegratorRTWStateStorageClass=Auto  FilterContinuousStateAttributes=''  FilterStateMustResolveToSignalObject=off  FilterRTWStateStorageClass=Auto  DifferentiatorICPrevScaledInput=0  DifferentiatorOutMin=[]  DifferentiatorOutMax=[]  FilterDiffOutCoefMin=[]  FilterDiffOutCoefMax=[]  SumDenOutMin=[]  SumDenOutMax=[]  SumNumOutMin=[]  SumNumOutMax=[]  ReciprocalOutMin=[]  ReciprocalOutMax=[]  DivideOutMin=[]  DivideOutMax=[]  TunerSelectOption=Transfer Function Based (PID Tuner App)
  PID Controller (2DOF)6 : simulink/Continuous/PID Controller (2DOF)  Controller=PID  TimeDomain=Discrete-time  SampleTime=-1  IntegratorMethod=Forward Euler  FilterMethod=Forward Euler  Form=Parallel  UseFilter=on  ControllerParametersSource=internal  P=0.3  I=0.08  D=0  N=100  b=1  c=1  InitialConditionSource=internal  InitialConditionForIntegrator=0  InitialConditionForFilter=0  ExternalReset=none  LimitOutput=off  UpperSaturationLimit=inf  LowerSaturationLimit=-inf  LinearizeAsGain=on  AntiWindupMode=none  Kb=1  TrackingMode=off  Kt=1  PParamMin=[]  PParamMax=[]  IParamMin=[]  IParamMax=[]  DParamMin=[]  DParamMax=[]  NParamMin=[]  NParamMax=[]  bParamMin=[]  bParamMax=[]  cParamMin=[]  cParamMax=[]  KbParamMin=[]  KbParamMax=[]  KtParamMin=[]  KtParamMax=[]  POutMin=[]  POutMax=[]  IOutMin=[]  IOutMax=[]  DOutMin=[]  DOutMax=[]  NOutMin=[]  NOutMax=[]  bOutMin=[]  bOutMax=[]  cOutMin=[]  cOutMax=[]  KbOutMin=[]  KbOutMax=[]  KtOutMin=[]  KtOutMax=[]  IntegratorOutMin=[]  IntegratorOutMax=[]  FilterOutMin=[]  FilterOutMax=[]  SumOutMin=[]  SumOutMax=[]  Sum1OutMin=[]  Sum1OutMax=[]  Sum2OutMin=[]  Sum2OutMax=[]  Sum3OutMin=[]  Sum3OutMax=[]  SumI1OutMin=[]  SumI1OutMax=[]  SumI2OutMin=[]  SumI2OutMax=[]  SumI3OutMin=[]  SumI3OutMax=[]  SumDOutMin=[]  SumDOutMax=[]  SaturationOutMin=[]  SaturationOutMax=[]  IntegratorContinuousStateAttributes=''  IntegratorStateMustResolveToSignalObject=off  IntegratorRTWStateStorageClass=Auto  FilterContinuousStateAttributes=''  FilterStateMustResolveToSignalObject=off  FilterRTWStateStorageClass=Auto  DifferentiatorICPrevScaledInput=0  DifferentiatorOutMin=[]  DifferentiatorOutMax=[]  FilterDiffOutCoefMin=[]  FilterDiffOutCoefMax=[]  SumDenOutMin=[]  SumDenOutMax=[]  SumNumOutMin=[]  SumNumOutMax=[]  ReciprocalOutMin=[]  ReciprocalOutMax=[]  DivideOutMin=[]  DivideOutMax=[]  TunerSelectOption=Transfer Function Based (PID Tuner App)
  PID Controller (2DOF)7 : simulink/Continuous/PID Controller (2DOF)  Controller=PID  TimeDomain=Discrete-time  SampleTime=-1  IntegratorMethod=Forward Euler  FilterMethod=Forward Euler  Form=Parallel  UseFilter=on  ControllerParametersSource=internal  P=2  I=0.2  D=2  N=100  b=1  c=1  InitialConditionSource=internal  InitialConditionForIntegrator=0  InitialConditionForFilter=0  ExternalReset=none  LimitOutput=off  UpperSaturationLimit=inf  LowerSaturationLimit=-inf  LinearizeAsGain=on  AntiWindupMode=none  Kb=1  TrackingMode=off  Kt=1  PParamMin=[]  PParamMax=[]  IParamMin=[]  IParamMax=[]  DParamMin=[]  DParamMax=[]  NParamMin=[]  NParamMax=[]  bParamMin=[]  bParamMax=[]  cParamMin=[]  cParamMax=[]  KbParamMin=[]  KbParamMax=[]  KtParamMin=[]  KtParamMax=[]  POutMin=[]  POutMax=[]  IOutMin=[]  IOutMax=[]  DOutMin=[]  DOutMax=[]  NOutMin=[]  NOutMax=[]  bOutMin=[]  bOutMax=[]  cOutMin=[]  cOutMax=[]  KbOutMin=[]  KbOutMax=[]  KtOutMin=[]  KtOutMax=[]  IntegratorOutMin=[]  IntegratorOutMax=[]  FilterOutMin=[]  FilterOutMax=[]  SumOutMin=[]  SumOutMax=[]  Sum1OutMin=[]  Sum1OutMax=[]  Sum2OutMin=[]  Sum2OutMax=[]  Sum3OutMin=[]  Sum3OutMax=[]  SumI1OutMin=[]  SumI1OutMax=[]  SumI2OutMin=[]  SumI2OutMax=[]  SumI3OutMin=[]  SumI3OutMax=[]  SumDOutMin=[]  SumDOutMax=[]  SaturationOutMin=[]  SaturationOutMax=[]  IntegratorContinuousStateAttributes=''  IntegratorStateMustResolveToSignalObject=off  IntegratorRTWStateStorageClass=Auto  FilterContinuousStateAttributes=''  FilterStateMustResolveToSignalObject=off  FilterRTWStateStorageClass=Auto  DifferentiatorICPrevScaledInput=0  DifferentiatorOutMin=[]  DifferentiatorOutMax=[]  FilterDiffOutCoefMin=[]  FilterDiffOutCoefMax=[]  SumDenOutMin=[]  SumDenOutMax=[]  SumNumOutMin=[]  SumNumOutMax=[]  ReciprocalOutMin=[]  ReciprocalOutMax=[]  DivideOutMin=[]  DivideOutMax=[]  TunerSelectOption=Transfer Function Based (PID Tuner App)
  Saturation : Saturate  UpperLimit=9.788  LowerLimit=-9.788
  Scope : Scope  NumInputPorts=2
  Signal Builder : Subsystem  Tag=STV Subsys  LoadFcn=sigbuilder_block('load');  StartFcn=sigbuilder_block('start');  StopFcn=sigbuilder_block('stop');  ClipboardFcn=sigbuilder_block('clipboard');  mask(Sigbuilder block){tuvar=[0:10]}
      mask help: Simulink:masks:SigbuilderBlock_MD
      mask init:
      | if ~strcmp(get_param(bdroot(gcbh),'SimulationStatus'),'stopped') tuvar = sigbuilder_block('maskInit'); end
      settings: CopyFcn=sigbuilder_block('copy');  DeleteFcn=sigbuilder_block('delete');  ModelCloseFcn=sigbuilder_block('modelClose');  PreSaveFcn=sigbuilder_block('preSave');  PauseFcn=sigbuilder_block('pause');  ContinueFcn=sigbuilder_block('continue');  NameChangeFcn=sigbuilder_block('namechange');  OpenFcn=sigbuilder_block('open',[5.5 30 949 419 ]);  CloseFcn=sigbuilder_block('close');
      mask Display: plot(0, 0, 100, 100,[2, 2, 32, 32, 2], [68, 8, 8, 68, 68],[32, 2], [38, 38], [32, 19, 2],[53, 60, 44], [32, 17, 17, 2],[16, 16, 31, 31]);txt = getActiveGroup(gcbh);text(2, 100, txt,'verticalAlignment', 'top');
  Sine Wave : Sin  Amplitude=0.2  Frequency=2*pi*1  SampleTime=0.01
  Subsystem : Subsystem
  Sum : Sum  Inputs=|+-
  Sum1 : Sum  Inputs=|+-
  Terminator2 : Terminator
  Terminator3 : Terminator
  Unit Delay1 : UnitDelay  SampleTime=-1
  gyro : Subsystem
  rate_d : Demux  Outputs=3
  舵面分配 : Subsystem
  ActuatorsBus : Outport  OutDataTypeStr=Bus: ActuatorsBus
  wires:
  PID Controller/1 -> Mux/3
  Bus Selector/3 -> Sum/1  "<yaw_cmd>"
  Demux/3 -> Sum/2
  PID Controller (2DOF)7/1 -> Saturation/1
  Bus Selector/2 -> PID Controller (2DOF)1/1  "<pitch_cmd>"
  Bus Selector1/2 -> Demux1/1  "<Omega_body>"
  Bus Selector1/1 -> Demux/1  "<<Euler>>"
  Sum/1 -> MATLAB Function1/1(u)
  PID Controller (2DOF)/1 -> Mux/1
  Demux3/2 -> Terminator2/1
  Demux/2 -> PID Controller (2DOF)1/2, Mux/5, Subsystem/1(In1)
  Demux1/2 -> PID Controller (2DOF)5/2, gyro/4(q)
  rate_d/3 -> PID Controller (2DOF)6/1
  PID Controller (2DOF)1/1 -> Mux/2
  Demux1/3 -> PID Controller (2DOF)6/2
  MATLAB Function1/1(y) -> PID Controller/1
  Demux3/1 -> Terminator3/1
  rate_d/2 -> PID Controller (2DOF)5/1
  rate_d/1 -> Sum1/1
  Mux/1 -> MATLAB Function/1(u)
  Command/1 -> Bus Selector/1
  Bus Creator/1 -> ActuatorsBus/1  "ActuatorsBus"
  Constant1/1 -> N-Sample Switch/1
  Subsystem/1(speed) -> N-Sample Switch/2  "speed"
  N-Sample Switch/1 -> Bus Creator/5, gyro/6(speed)  "speed"
  Demux3/3 -> PID Controller (2DOF)7/2  "h"
  MATLAB Function/1(y) -> rate_d/1
  States/1 -> Unit Delay1/1
  Unit Delay1/1 -> Bus Selector1/1
  Add/1 -> Subsystem/3(In3)  "a_t"
  Constant/1 -> Add/1
  Sum1/1 -> Discrete PID Controller/1
  Sine Wave/1 -> Scope/1
  Bus Selector/1 -> PID Controller (2DOF)/1  "<roll_cmd>"
  Saturation/1 -> Add/2
  Demux/1 -> Scope/2, PID Controller (2DOF)/2, Subsystem/2(In2), Mux/4
  Demux1/1 -> Sum1/2, gyro/2(p)
  舵面分配/1(c1) -> Bus Creator/1
  舵面分配/2(c2) -> Bus Creator/2
  舵面分配/3(c3) -> Bus Creator/3
  Bus Selector1/3 -> Demux3/1  "<X_ned>"
  Bus Selector/4 -> PID Controller (2DOF)7/1  "<throttle_cmd>"
  ? -> ?  "反馈"
  gyro/1(u_1) -> 舵面分配/1(u_1)
  gyro/2(u_2) -> 舵面分配/2(u_2)
  gyro/3(u_3) -> 舵面分配/3(u_3)
  Discrete PID Controller/1 -> gyro/1(u_p)
  PID Controller (2DOF)5/1 -> gyro/3(u_q)
  PID Controller (2DOF)6/1 -> gyro/5(u_r)
  舵面分配/4(c4) -> Bus Creator/4
